simulink model "chris_1R_setpoint"  (R2016b)
settings: Solver=FixedStepDiscrete  StartTime=0.0  StopTime=15  FixedStep=0.1  MaxStep=0.1  RelTol=1e-3
libraries: simulink x1, realtime_pacer_lib x1
settings Model: Creator=RSL  LastModifiedBy=RSL

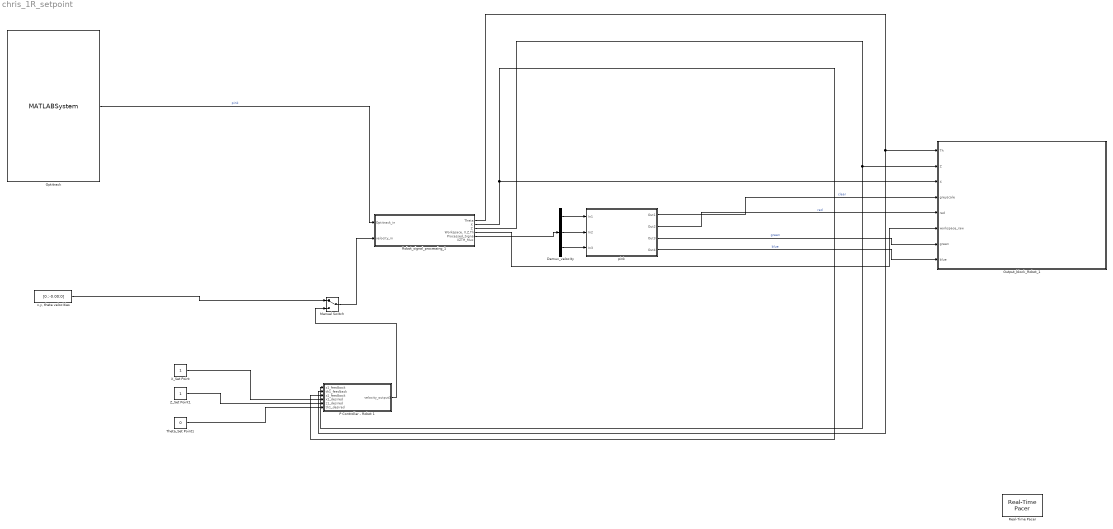
== system chris_1R_setpoint ==
  Demux_velocity : Demux  Outputs=3
  Manual Switch : ManualSwitch
  Optitrack : MATLABSystem  System=OptiTrackRigidBody  coordinateTransformationMatrix=[ 1, 0, 0; 0, 0, 1; 0, -1, 0 ]  rigidBodyNames={ 'pink'}  orientationFormat=Euler angles  debug=on  natNetHostAddress=127.0.0.1  natNetClientAddress=127.0.0.1  dllPath=C:\DecaMATLAB\NatNetSDK\lib\x64\NatNetML.dll  unicast=off
      mask Type: OptiTrackRigidBody
      mask Display:
      | disp('OptiTrackRigidBody');
      | port_label('output',1,'pink');
  Output_block_Robot_1 : Subsystem
  P Controller - Robot 1 : Subsystem
  Real-Time Pacer : realtime_pacer_lib/Real-Time Pacer  simTimePerRealTime=1
  Robot_signal_processing_1 : Subsystem
  "Theta_Set Point1 " : Constant  Value=0
  X_Set Point : Constant
  Z_Set Point1 : Constant
  pink : Subsystem  mask(DecabotMask){robotName=pink, decabotHelper=localhost, robotAddress=, useDataTurbine=off, useDirectSocket=on, debug=off}
      mask prompts: robotName "Robot name:"; decabotHelper "DecabotHelper/DataTurbine server:"; robotAddress "Robot network address (optional):"; useDataTurbine "Use DataTurbine"; useDirectSocket "Use direct robot TCP connection"; debug "Log debug messages"
      mask help: This is a masked subsystem that contains a Decabot block for bidirectional communication with a decabot over a direct TCP socket connection.
      mask init:
      | robotName = 'Nobody';
      | decabotHelper = 'localhost';
      | robotAddress = '';
      | useDataTurbine = true;
      | debug = true;
      mask TypeOptions robotName: decabot/robotName
      mask Callback robotName:
      | try
      |     set_param( gcb( ), 'Name', get_param( gcb( ), 'robotName' ) );
      | end
      mask TypeOptions decabotHelper: decabot/decabotHelper
      mask TypeOptions robotAddress: decabot/robotAddress
      mask TypeOptions useDataTurbine: decabot/useDataTurbine
      mask TypeOptions useDirectSocket: decabot/useDirectSocket
      mask TypeOptions debug: decabot/debug
      mask Display:
      | disp( [get_param( gcb( ), 'robotName' ) '\n\nDH: ' get_param( gcb( ), 'decabotHelper' ) ] );
      | 
      | port_label('input',1,'x_vel');
      | port_label('input',2,'y_vel');
      | port_label('input',3,'t_vel');
      | 
      | port_label('output',1,'clear');
      | port_label('output',2,'red');
      | port_label('output',3,'green');
      | port_label('output',4,'blue');
  "x,y, theta velocities" : Constant  Value=[0.;-0.00;0]
  wires:
  Demux_velocity/3 -> pink/3(In3)
  Demux_velocity/1 -> pink/1(In1)
  Demux_velocity/2 -> pink/2(In2)
  "x,y, theta velocities"/1 -> Manual Switch/1
  X_Set Point/1 -> P Controller - Robot 1/4(x1_desired)
  Z_Set Point1/1 -> P Controller - Robot 1/5(z1_desired)
  "Theta_Set Point1 "/1 -> P Controller - Robot 1/6(th1_desired)
  P Controller - Robot 1/1(velocity_output1) -> Manual Switch/2
  Robot_signal_processing_1/1(Theta) -> P Controller - Robot 1/2(th1_feedback), Output_block_Robot_1/1(Th)
  Robot_signal_processing_1/3(Z) -> Output_block_Robot_1/2(Z), P Controller - Robot 1/1(z1_feedback)
  Robot_signal_processing_1/2(X) -> P Controller - Robot 1/3(x1_feedback), Output_block_Robot_1/3(X)
  Optitrack/1 -> Robot_signal_processing_1/1(Optitrack_in)  "pink"
  Manual Switch/1 -> Robot_signal_processing_1/2(velocity_in)
  Robot_signal_processing_1/5(Processed_Signal) -> Demux_velocity/1
  pink/1(Out1) -> Output_block_Robot_1/4(greyscale)  "clear"
  pink/2(Out2) -> Output_block_Robot_1/5(red)  "red"
  Robot_signal_processing_1/4("Workspace, X,Z,Th") -> Output_block_Robot_1/6(workspace_raw)
  pink/3(Out3) -> Output_block_Robot_1/7(green)  "green"
  pink/4(Out4) -> Output_block_Robot_1/8(blue)  "blue"

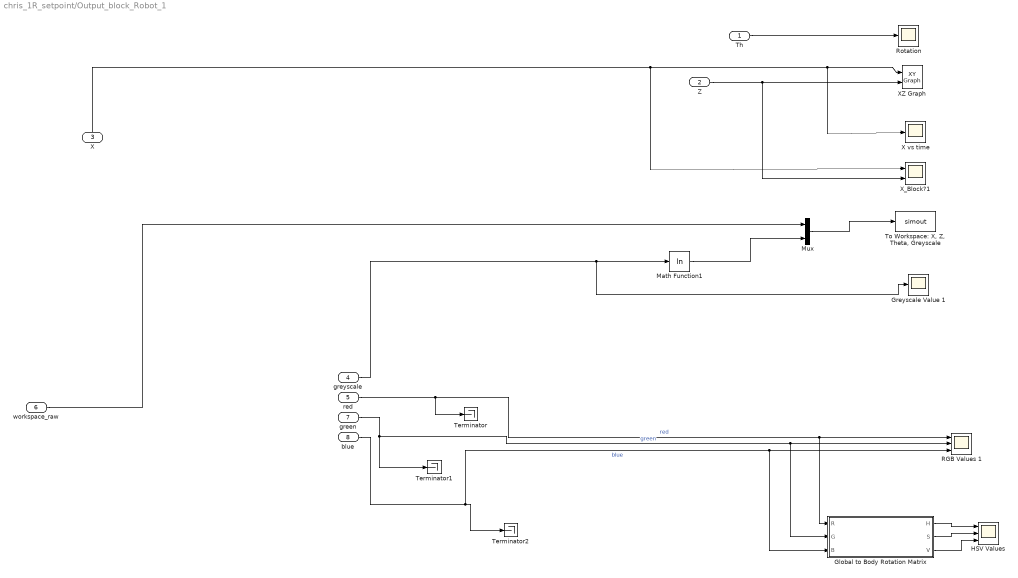
== system chris_1R_setpoint/Output_block_Robot_1 ==
  Th : Inport
  Z : Inport  Port=2
  X : Inport  Port=3
  greyscale : Inport  Port=4
  red : Inport  Port=5
  workspace_raw : Inport  Port=6
  green : Inport  Port=7
  blue : Inport  Port=8
  Global to Body Rotation Matrix : MATLAB Function  TreatAsAtomicUnit=on
  Greyscale Value 1 : Scope
  HSV Values : Scope  NumInputPorts=3
  Math Function1 : Math  Operator=log  SaturateOnIntegerOverflow=on
  Mux : Mux  Inputs=2
  "RGB Values 1 " : Scope  NumInputPorts=3
  Rotation : Scope
  Terminator : Terminator
  Terminator1 : Terminator
  Terminator2 : Terminator
  "To Workspace: X, Z, Theta, Greyscale" : ToWorkspace  VariableName=simout  SaveFormat=Timeseries  SampleTime=-1
  X vs time : Scope
  XZ Graph : simulink/Sinks/XY Graph  xmin=-1  xmax=10  ymin=-1  ymax=10  st=-1
  X_Block?1 : Scope  NumInputPorts=2
  wires:
  Th/1 -> Rotation/1
  X/1 -> X_Block?1/1, X vs time/1, XZ Graph/1
  Z/1 -> X_Block?1/2, XZ Graph/2
  workspace_raw/1 -> Mux/1
  red/1 -> Global to Body Rotation Matrix/1(R), "RGB Values 1 "/1, Terminator/1  "red"
  blue/1 -> Global to Body Rotation Matrix/3(B), "RGB Values 1 "/3, Terminator2/1  "blue"
  greyscale/1 -> Greyscale Value 1/1, Math Function1/1
  Mux/1 -> "To Workspace: X, Z, Theta, Greyscale"/1
  Math Function1/1 -> Mux/2
  green/1 -> Terminator1/1, Global to Body Rotation Matrix/2(G), "RGB Values 1 "/2  "green"
  Global to Body Rotation Matrix/1(H) -> HSV Values/1
  Global to Body Rotation Matrix/2(S) -> HSV Values/2
  Global to Body Rotation Matrix/3(V) -> HSV Values/3

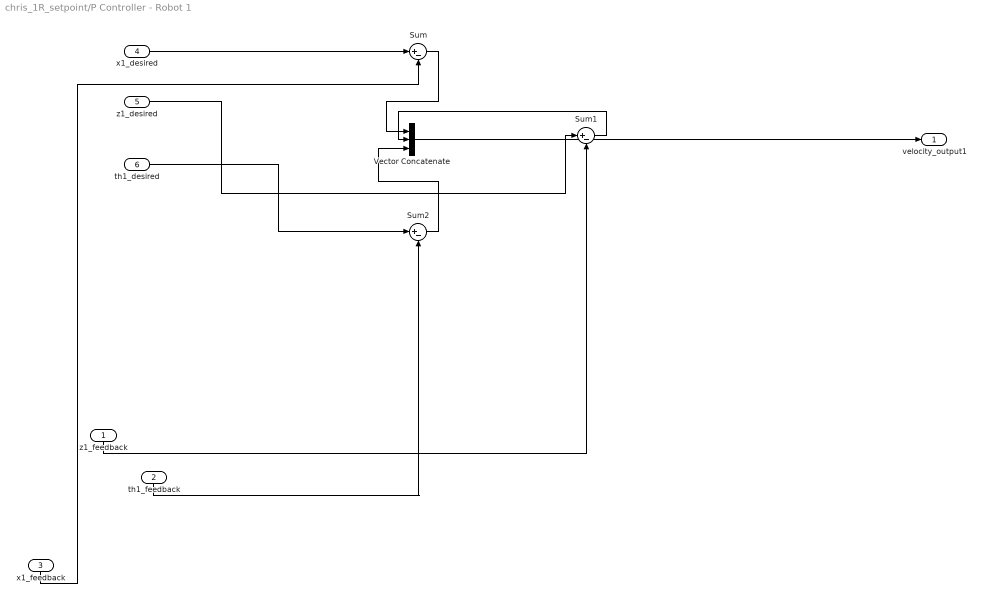
== system chris_1R_setpoint/P Controller - Robot 1 ==
  z1_feedback : Inport
  th1_feedback : Inport  Port=2
  x1_feedback : Inport  Port=3
  x1_desired : Inport  Port=4
  z1_desired : Inport  Port=5
  th1_desired : Inport  Port=6
  Sum : Sum  Inputs=|+-
  Sum1 : Sum  Inputs=|+-
  Sum2 : Sum  Inputs=|+-
  Vector Concatenate : Concatenate  NumInputs=3
  velocity_output1 : Outport
  wires:
  Vector Concatenate/1 -> velocity_output1/1
  x1_desired/1 -> Sum/1
  Sum/1 -> Vector Concatenate/1
  th1_feedback/1 -> Sum2/2
  x1_feedback/1 -> Sum/2
  z1_feedback/1 -> Sum1/2
  Sum2/1 -> Vector Concatenate/3
  th1_desired/1 -> Sum2/1
  Sum1/1 -> Vector Concatenate/2
  z1_desired/1 -> Sum1/1

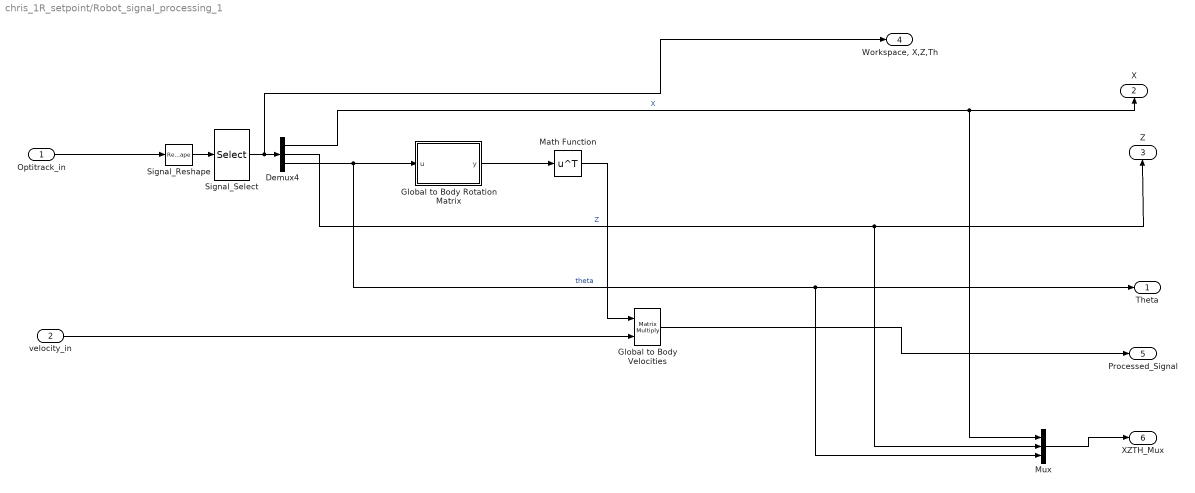
== system chris_1R_setpoint/Robot_signal_processing_1 ==
  Optitrack_in : Inport
  velocity_in : Inport  Port=2
  Demux4 : Demux  Outputs=3
  Global to Body Velocities : Product  Multiplication=Matrix(*)
  Global to Body Rotation Matrix : MATLAB Function  TreatAsAtomicUnit=on
  Math Function : Math  Operator=transpose  SaturateOnIntegerOverflow=on
  Mux : Mux  Inputs=3
  Signal_Reshape : Reshape  OutputDimensions=6
  Signal_Select : Selector  InputPortWidth=6  IndexOptions=Index vector (dialog)  Indices=[1 2 6]  OutputSizes=1
  Theta : Outport
  X : Outport  Port=2
  Z : Outport  Port=3
  "Workspace, X,Z,Th" : Outport  Port=4
  Processed_Signal : Outport  Port=5
  XZTH_Mux : Outport  Port=6
  wires:
  Demux4/1 -> Mux/1, X/1  "X"
  Demux4/3 -> Mux/3, Theta/1, Global to Body Rotation Matrix/1(u)  "theta"
  Demux4/2 -> Mux/2, Z/1  "Z"
  Global to Body Velocities/1 -> Processed_Signal/1
  Signal_Reshape/1 -> Signal_Select/1
  velocity_in/1 -> Global to Body Velocities/2
  Optitrack_in/1 -> Signal_Reshape/1
  Global to Body Rotation Matrix/1(y) -> Math Function/1
  Signal_Select/1 -> "Workspace, X,Z,Th"/1, Demux4/1
  Math Function/1 -> Global to Body Velocities/1
  Mux/1 -> XZTH_Mux/1

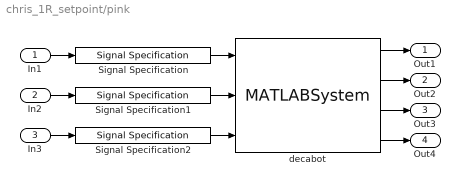
== system chris_1R_setpoint/pink ==
  In1 : Inport
  In2 : Inport  Port=2
  In3 : Inport  Port=3
  Signal Specification : SignalSpecification  OutDataTypeStr=double  Dimensions=1
  Signal Specification1 : SignalSpecification  OutDataTypeStr=double  Dimensions=1
  Signal Specification2 : SignalSpecification  OutDataTypeStr=double  Dimensions=1
  decabot : MATLABSystem  System=Decabot  robotName=pink  decabotHelper=localhost  useDataTurbine=off  useDirectSocket=on  debug=off
      mask Type: Decabot
      mask Display:
      | disp('pink\n\nDH: localhost');
      | port_label('input',1,'x_vel');
      | port_label('input',2,'y_vel');
      | port_label('input',3,'t_vel');
      | port_label('output',1,'clear');
      | port_label('output',2,'red');
      | port_label('output',3,'green');
      | port_label('output',4,'blue');
  Out1 : Outport
  Out2 : Outport  Port=2
  Out3 : Outport  Port=3
  Out4 : Outport  Port=4
  wires:
  Signal Specification2/1 -> decabot/3
  Signal Specification1/1 -> decabot/2
  Signal Specification/1 -> decabot/1
  In2/1 -> Signal Specification1/1
  decabot/4 -> Out4/1
  decabot/1 -> Out1/1
  decabot/3 -> Out3/1
  decabot/2 -> Out2/1
  In1/1 -> Signal Specification/1
  In3/1 -> Signal Specification2/1

== matlab function chris_1R_setpoint/Output_block_Robot_1/Global to Body Rotation Matrix ==
  data: R input; H output; G input; B input; S output; V output
function [H, S, V]= rgb2hsv_func(R, G, B)
  % Clip RGB values to be within the range [100, 900]
  R = max(min(R, 1200), 100);
  G = max(min(G, 1200), 100);
  B = max(min(B, 1200), 100);

  % Normalize RGB to [0, 1]
  R = (R - 100) / 800; 
  G = (G - 100) / 800;
  B = (B - 100) / 800;

  Cmax = max(max(R, G), B);
  Cmin = min(min(R, G), B);
  delta = Cmax - Cmin;

  H = zeros(size(R));
  S = zeros(size(R));
  V = Cmax;

  % Calculate Hue
  ind = find(delta ~= 0); 
  r_ind = find((Cmax == R) & (delta ~= 0));
  g_ind = find((Cmax == G) & (delta ~= 0));
  b_ind = find((Cmax == B) & (delta ~= 0));

  H(r_ind) = 60 * mod((G(r_ind) - B(r_ind)) ./ delta(r_ind), 6);
  H(g_ind) = 60 * (((B(g_ind) - R(g_ind)) ./ delta(g_ind)) + 2);
  H(b_ind) = 60 * (((R(b_ind) - G(b_ind)) ./ delta(b_ind)) + 4);

  H = H / 360;

  % Calculate Saturation
  S(ind) = delta(ind) ./ Cmax(ind);

end

== matlab function chris_1R_setpoint/Robot_signal_processing_1/Global to Body Rotation Matrix ==
  data: u input; y output
function y = fcn(u)

y = [cos(u) -sin(u) 0; sin(u) cos(u) 0; 0 0 1];
